simulink model "fadob_simulink"  (R2026a)
settings: Solver=ode3  StartTime=0  StopTime=3  FixedStep=1e-4
settings Model: Creator=hzldx  LastModifiedBy=hzldx

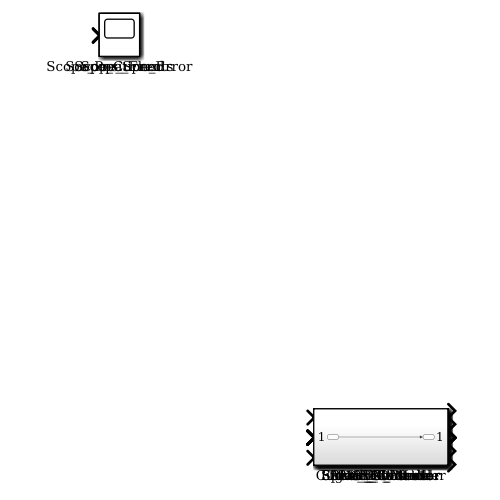
[thumbnail: Simulink's stored preview of the top-level diagram]
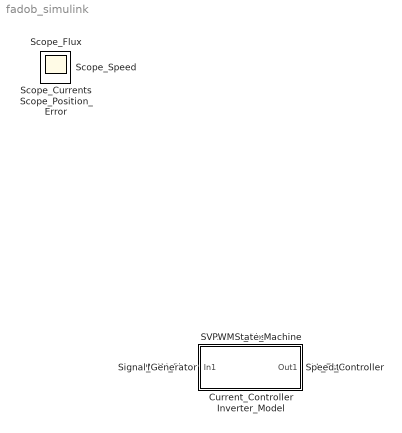
== system fadob_simulink ==
  Current_Controller : Subsystem
  FADOB_Observer : Subsystem
  Inverter_Model : Subsystem
  PLL_Estimator : Subsystem
  PMSM_Plant : Subsystem
  SVPWM : Subsystem
  Scope_Currents : Scope
  Scope_Flux : Scope
  Scope_Position_Error : Scope
  Scope_Speed : Scope
  Signal_Generator : Subsystem
  Speed_Controller : Subsystem
  State_Machine : Subsystem

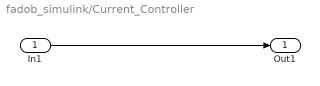
== system fadob_simulink/Current_Controller ==
  In1 : Inport
  Out1 : Outport
  wires:
  In1/1 -> Out1/1

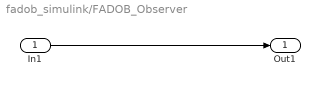
== system fadob_simulink/FADOB_Observer ==
  In1 : Inport
  Out1 : Outport
  wires:
  In1/1 -> Out1/1

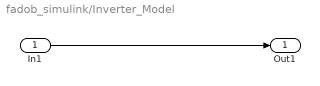
== system fadob_simulink/Inverter_Model ==
  In1 : Inport
  Out1 : Outport
  wires:
  In1/1 -> Out1/1

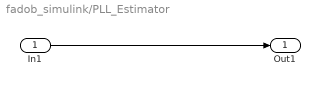
== system fadob_simulink/PLL_Estimator ==
  In1 : Inport
  Out1 : Outport
  wires:
  In1/1 -> Out1/1

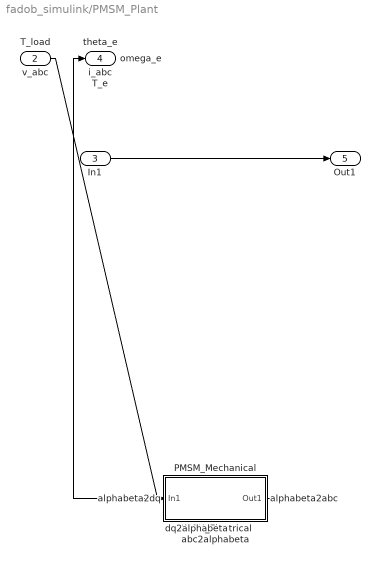
== system fadob_simulink/PMSM_Plant ==
  v_abc : Inport
  T_load : Inport  Port=2
  In1 : Inport  Port=3
  PMSM_Electrical : Subsystem
  PMSM_Mechanical : Subsystem
  abc2alphabeta : Subsystem
  alphabeta2abc : Subsystem
  alphabeta2dq : Subsystem
  dq2alphabeta : Subsystem
  i_abc : Outport
  theta_e : Outport  Port=2
  omega_e : Outport  Port=3
  T_e : Outport  Port=4
  Out1 : Outport  Port=5
  wires:
  In1/1 -> Out1/1
  v_abc/1 -> abc2alphabeta/1(In1)
  abc2alphabeta/1(Out1) -> ?
  ? -> PMSM_Electrical/1(In1)
  PMSM_Electrical/1(Out1) -> dq2alphabeta/1(In1)
  dq2alphabeta/1(Out1) -> alphabeta2abc/1(In1)
  alphabeta2abc/1(Out1) -> i_abc/1
  T_load/1 -> PMSM_Mechanical/1(In1)

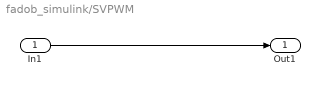
== system fadob_simulink/SVPWM ==
  In1 : Inport
  Out1 : Outport
  wires:
  In1/1 -> Out1/1

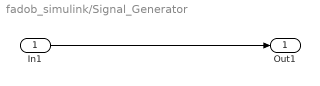
== system fadob_simulink/Signal_Generator ==
  In1 : Inport
  Out1 : Outport
  wires:
  In1/1 -> Out1/1

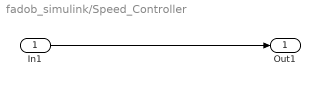
== system fadob_simulink/Speed_Controller ==
  In1 : Inport
  Out1 : Outport
  wires:
  In1/1 -> Out1/1

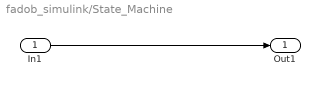
== system fadob_simulink/State_Machine ==
  In1 : Inport
  Out1 : Outport
  wires:
  In1/1 -> Out1/1

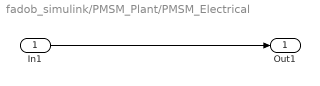
== system fadob_simulink/PMSM_Plant/PMSM_Electrical ==
  In1 : Inport
  Out1 : Outport
  wires:
  In1/1 -> Out1/1

== system fadob_simulink/PMSM_Plant/PMSM_Mechanical ==
  In1 : Inport
  Out1 : Outport
  wires:
  In1/1 -> Out1/1

== system fadob_simulink/PMSM_Plant/abc2alphabeta ==
  In1 : Inport
  Out1 : Outport
  wires:
  In1/1 -> Out1/1

== system fadob_simulink/PMSM_Plant/alphabeta2abc ==
  In1 : Inport
  Out1 : Outport
  wires:
  In1/1 -> Out1/1

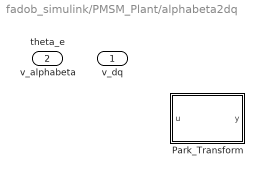
== system fadob_simulink/PMSM_Plant/alphabeta2dq ==
  v_alphabeta : Inport
  theta_e : Inport  Port=2
  Park_Transform : MATLAB Function  TreatAsAtomicUnit=on
  v_dq : Outport
  wires:
  ? -> ?

== system fadob_simulink/PMSM_Plant/dq2alphabeta ==
  In1 : Inport
  Out1 : Outport
  wires:
  In1/1 -> Out1/1

== matlab function fadob_simulink/PMSM_Plant/alphabeta2dq/Park_Transform ==
  data: u input; y output
function y = fcn(u)

y = u;
